simulink model "PX4OutputMappingBicycleRover"  (R2026a)
settings: Solver=ode4  FixedStep=stepSize_s
undefined symbols (not defined in the file): ServosCommandBicycleRoverBus
settings Model: Creator=Edison Altamirano  LastModifiedBy=Edison Altamirano

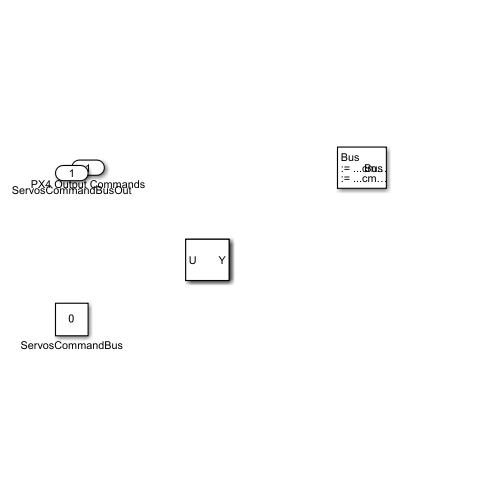
[thumbnail: Simulink's stored preview of the top-level diagram]
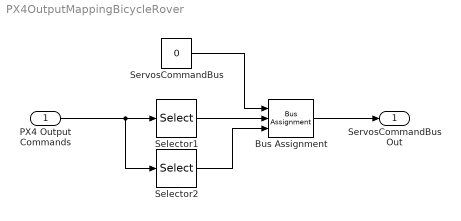
== system PX4OutputMappingBicycleRover ==
  PX4 Output Commands : Inport  PortDimensions=16
  Bus Assignment : BusAssignment  AssignedSignals=ServosCommandBicycleRoverBus.cmdSteering_nd,ServosCommandBicycleRoverBus.cmdThrottle_nd
  Selector1 : Selector  InputPortWidth=16  IndexOptions=Index vector (dialog)  Indices=1  OutputSizes=1
  Selector2 : Selector  InputPortWidth=16  IndexOptions=Index vector (dialog)  Indices=2  OutputSizes=1
  ServosCommandBus : Constant  Value=0  OutDataTypeStr=Bus: ServosCommandBus
  ServosCommandBusOut : Outport  OutDataTypeStr=Bus: ServosCommandBus
  wires:
  Selector1/1 -> Bus Assignment/2
  PX4 Output Commands/1 -> Selector1/1, Selector2/1
  Bus Assignment/1 -> ServosCommandBusOut/1
  ServosCommandBus/1 -> Bus Assignment/1
  Selector2/1 -> Bus Assignment/3
